simulink model "Space_Shuttle"  (R2023a)
settings: Solver=ode45  StartTime=0.0  StopTime=1000  RelTol=1e-4
undefined symbols (not defined in the file or in its folder): Earth, WGS84
libraries: simulink_extras x4, slpidlib x3, simulink x3, aerolibadyn x1, aerolibatmos2 x1, aerolib6dof2 x1
settings Model: PauseTimes=0  Creator=francesconuzzo  LastModifiedBy=francesconuzzo

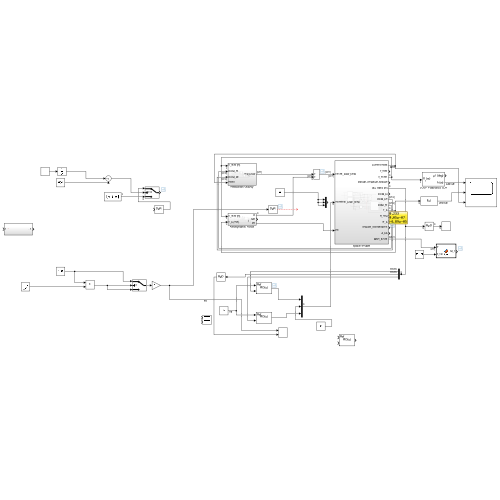
[thumbnail: Simulink's stored preview of the top-level diagram]
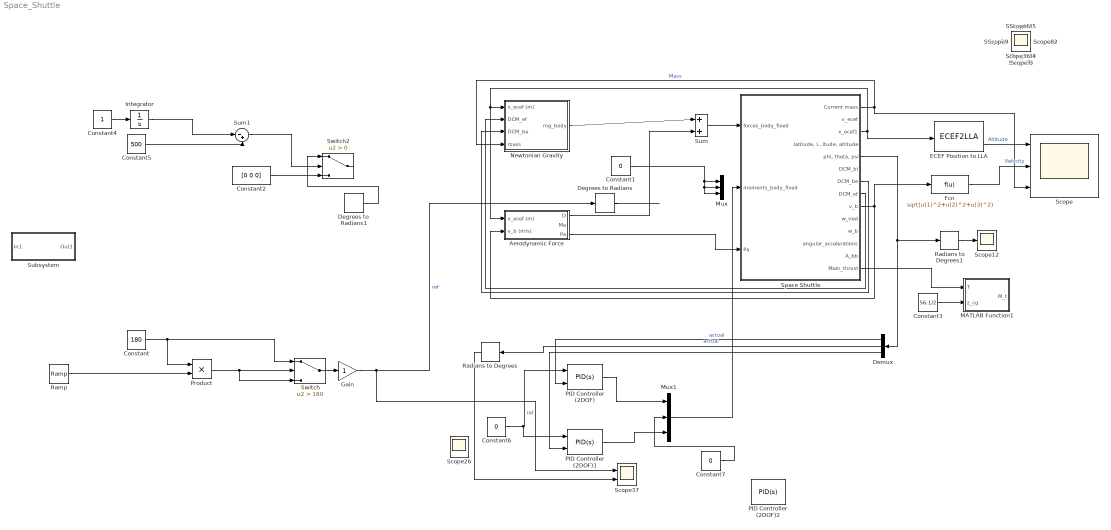
== system Space_Shuttle ==
  Aerodynamic Force : Subsystem
  Constant : Constant  Value=180
  Constant1 : Constant  Value=0
  Constant2 : Constant  Value=[0 0 0]
  Constant3 : Constant  Value=56.1/2
  Constant4 : Constant
  Constant5 : Constant  Value=500
  Constant6 : Constant  Value=0
  Constant7 : Constant  Value=0
  Degrees to Radians : simulink_extras/Transformations/Degrees to Radians
  Degrees to Radians1 : simulink_extras/Transformations/Degrees to Radians
  Demux : Demux  Outputs=3
  ECEF Position to LLA : ECEF2LLA
  Fcn : Fcn  Expr=sqrt(u(1)^2+u(2)^2+u(3)^2)
  Gain : Gain
  Integrator : Integrator
  MATLAB Function1 : MATLAB Function  TreatAsAtomicUnit=on
  Mux : Mux  Inputs=3
  Mux1 : Mux  Inputs=3
  Newtonian Gravity : Subsystem
  PID Controller (2DOF) : slpidlib/PID Controller (2DOF)  Controller=PID  Form=Parallel  TimeDomain=Continuous-time  UseExternalTs=off  SampleTime=-1  IntegratorMethod=Forward Euler  FilterMethod=Forward Euler  ControllerParametersSource=internal  P=1  I=0  UseKiTs=off  D=0  N=100  UseFilter=on  b=0  c=0  TunerSelectOption=Transfer Function Based (PID Tuner App)  InitialConditionSource=internal  InitialConditionForIntegrator=0  InitialConditionForFilter=0  DifferentiatorICPrevScaledInput=0  ExternalReset=none  TrackingMode=off  Kt=1  LimitOutput=off  SatLimitsSource=internal  UpperSaturationLimit=inf  LowerSaturationLimit=-inf  LinearizeAsGain=on  AntiWindupMode=none  Kb=1  LimitIntegrator=off  UpperIntegratorSaturationLimit=inf  LowerIntegratorSaturationLimit=-inf  POutMin=[]  POutMax=[]  IOutMin=[]  IOutMax=[]  DOutMin=[]  DOutMax=[]  NOutMin=[]  NOutMax=[]  bOutMin=[]  bOutMax=[]  cOutMin=[]  cOutMax=[]  SumOutMin=[]  SumOutMax=[]  SaturationOutMin=[]  SaturationOutMax=[]  PParamMin=[]  PParamMax=[]  IParamMin=[]  IParamMax=[]  DParamMin=[]  DParamMax=[]  NParamMin=[]  NParamMax=[]  bParamMin=[]  bParamMax=[]  cParamMin=[]  cParamMax=[]  KbParamMin=[]  KbParamMax=[]  KtParamMin=[]  KtParamMax=[]  KbOutMin=[]  KbOutMax=[]  KtOutMin=[]  KtOutMax=[]  IntegratorOutMin=[]  IntegratorOutMax=[]  FilterOutMin=[]  FilterOutMax=[]  SumI1OutMin=[]  SumI1OutMax=[]  SumI2OutMin=[]  SumI2OutMax=[]  SumI3OutMin=[]  SumI3OutMax=[]  SumI4OutMin=[]  SumI4OutMax=[]  SumDOutMin=[]  SumDOutMax=[]  Sum1OutMin=[]  Sum1OutMax=[]  Sum2OutMin=[]  Sum2OutMax=[]  Sum3OutMin=[]  Sum3OutMax=[]  DifferentiatorOutMin=[]  DifferentiatorOutMax=[]  FilterDiffOutCoefMin=[]  FilterDiffOutCoefMax=[]  ReciprocalOutMin=[]  ReciprocalOutMax=[]  SumDenOutMin=[]  SumDenOutMax=[]  SumNumOutMin=[]  SumNumOutMax=[]  DivideOutMin=[]  DivideOutMax=[]  UdiffTsProdOutMin=[]  UdiffTsProdOutMax=[]  NTsProdOutMin=[]  NTsProdOutMax=[]  UintegralTsProdOutMin=[]  UintegralTsProdOutMax=[]  UngainTsProdOutMin=[]  UngainTsProdOutMax=[]  ClampingZeroOutDataTypeStr=Inherit: Inherit via back propagation  ClampingZeroOutMin=[]  ClampingZeroOutMax=[]  FilterDenConstantOutDataTypeStr=Inherit: Inherit via back propagation  FilterDenConstantOutMin=[]  FilterDenConstantOutMax=[]  PCopyOutDataTypeStr=Inherit: Inherit via back propagation  PCopyOutMin=[]  PCopyOutMax=[]  NCopyOutDataTypeStr=Inherit: Inherit via back propagation  NCopyOutMin=[]  NCopyOutMax=[]  IntegratorContinuousStateAttributes=''  IntegratorStateMustResolveToSignalObject=off  IntegratorRTWStateStorageClass=Auto  FilterContinuousStateAttributes=''  FilterStateMustResolveToSignalObject=off  FilterRTWStateStorageClass=Auto  ParallelPVariant=InternalParameters  IdealPVariant=Disabled  IVariant=InternalParameters  DVariant=InternalParameters  bVariant=InternalParameters  cVariant=InternalParameters  IntegratorVariant=Continuous  SatVariant=Disabled  AWVariant=Passthrough  PCopyVariant=Disabled  TRVariant=Disabled  FdbkBlocksVariant=Forward  IdealPFdbkVariant=Disabled  SatFdbkVariant=Disabled  DerivativeFilterVariant=ContFilter  NVariant=InternalParameters  NCopyVariant=Disabled  FilterICVariant=InternalICsFilter  IntegratorICVariant=InternalICs  ExternalResetVariant=Disabled  TRSumVariant=Passthrough  SumFdbkVariant=Disabled  SumVariant=Sum_PID  TsampFilterVariant=InternalTs  TsampNgainVariant=Passthrough  TsampIntegralVariant=Disabled_SignalSpec  ExternalSaturationOutDataTypeStr=Inherit: Same as second input
  PID Controller (2DOF)1 : slpidlib/PID Controller (2DOF)  Controller=PID  Form=Parallel  TimeDomain=Continuous-time  UseExternalTs=off  SampleTime=-1  IntegratorMethod=Forward Euler  FilterMethod=Forward Euler  ControllerParametersSource=internal  P=1  I=0  UseKiTs=off  D=0  N=100  UseFilter=on  b=0  c=0  TunerSelectOption=Transfer Function Based (PID Tuner App)  InitialConditionSource=internal  InitialConditionForIntegrator=0  InitialConditionForFilter=0  DifferentiatorICPrevScaledInput=0  ExternalReset=none  TrackingMode=off  Kt=1  LimitOutput=off  SatLimitsSource=internal  UpperSaturationLimit=inf  LowerSaturationLimit=-inf  LinearizeAsGain=on  AntiWindupMode=none  Kb=1  LimitIntegrator=off  UpperIntegratorSaturationLimit=inf  LowerIntegratorSaturationLimit=-inf  POutMin=[]  POutMax=[]  IOutMin=[]  IOutMax=[]  DOutMin=[]  DOutMax=[]  NOutMin=[]  NOutMax=[]  bOutMin=[]  bOutMax=[]  cOutMin=[]  cOutMax=[]  SumOutMin=[]  SumOutMax=[]  SaturationOutMin=[]  SaturationOutMax=[]  PParamMin=[]  PParamMax=[]  IParamMin=[]  IParamMax=[]  DParamMin=[]  DParamMax=[]  NParamMin=[]  NParamMax=[]  bParamMin=[]  bParamMax=[]  cParamMin=[]  cParamMax=[]  KbParamMin=[]  KbParamMax=[]  KtParamMin=[]  KtParamMax=[]  KbOutMin=[]  KbOutMax=[]  KtOutMin=[]  KtOutMax=[]  IntegratorOutMin=[]  IntegratorOutMax=[]  FilterOutMin=[]  FilterOutMax=[]  SumI1OutMin=[]  SumI1OutMax=[]  SumI2OutMin=[]  SumI2OutMax=[]  SumI3OutMin=[]  SumI3OutMax=[]  SumI4OutMin=[]  SumI4OutMax=[]  SumDOutMin=[]  SumDOutMax=[]  Sum1OutMin=[]  Sum1OutMax=[]  Sum2OutMin=[]  Sum2OutMax=[]  Sum3OutMin=[]  Sum3OutMax=[]  DifferentiatorOutMin=[]  DifferentiatorOutMax=[]  FilterDiffOutCoefMin=[]  FilterDiffOutCoefMax=[]  ReciprocalOutMin=[]  ReciprocalOutMax=[]  SumDenOutMin=[]  SumDenOutMax=[]  SumNumOutMin=[]  SumNumOutMax=[]  DivideOutMin=[]  DivideOutMax=[]  UdiffTsProdOutMin=[]  UdiffTsProdOutMax=[]  NTsProdOutMin=[]  NTsProdOutMax=[]  UintegralTsProdOutMin=[]  UintegralTsProdOutMax=[]  UngainTsProdOutMin=[]  UngainTsProdOutMax=[]  ClampingZeroOutDataTypeStr=Inherit: Inherit via back propagation  ClampingZeroOutMin=[]  ClampingZeroOutMax=[]  FilterDenConstantOutDataTypeStr=Inherit: Inherit via back propagation  FilterDenConstantOutMin=[]  FilterDenConstantOutMax=[]  PCopyOutDataTypeStr=Inherit: Inherit via back propagation  PCopyOutMin=[]  PCopyOutMax=[]  NCopyOutDataTypeStr=Inherit: Inherit via back propagation  NCopyOutMin=[]  NCopyOutMax=[]  IntegratorContinuousStateAttributes=''  IntegratorStateMustResolveToSignalObject=off  IntegratorRTWStateStorageClass=Auto  FilterContinuousStateAttributes=''  FilterStateMustResolveToSignalObject=off  FilterRTWStateStorageClass=Auto  ParallelPVariant=InternalParameters  IdealPVariant=Disabled  IVariant=InternalParameters  DVariant=InternalParameters  bVariant=InternalParameters  cVariant=InternalParameters  IntegratorVariant=Continuous  SatVariant=Disabled  AWVariant=Passthrough  PCopyVariant=Disabled  TRVariant=Disabled  FdbkBlocksVariant=Forward  IdealPFdbkVariant=Disabled  SatFdbkVariant=Disabled  DerivativeFilterVariant=ContFilter  NVariant=InternalParameters  NCopyVariant=Disabled  FilterICVariant=InternalICsFilter  IntegratorICVariant=InternalICs  ExternalResetVariant=Disabled  TRSumVariant=Passthrough  SumFdbkVariant=Disabled  SumVariant=Sum_PID  TsampFilterVariant=InternalTs  TsampNgainVariant=Passthrough  TsampIntegralVariant=Disabled_SignalSpec  ExternalSaturationOutDataTypeStr=Inherit: Same as second input
  PID Controller (2DOF)2 : slpidlib/PID Controller (2DOF)  Controller=PID  Form=Parallel  TimeDomain=Continuous-time  UseExternalTs=off  SampleTime=-1  IntegratorMethod=Forward Euler  FilterMethod=Forward Euler  ControllerParametersSource=internal  P=1  I=1  UseKiTs=off  D=0  N=100  UseFilter=on  b=1  c=1  TunerSelectOption=Transfer Function Based (PID Tuner App)  InitialConditionSource=internal  InitialConditionForIntegrator=0  InitialConditionForFilter=0  DifferentiatorICPrevScaledInput=0  ExternalReset=none  TrackingMode=off  Kt=1  LimitOutput=off  SatLimitsSource=internal  UpperSaturationLimit=inf  LowerSaturationLimit=-inf  LinearizeAsGain=on  AntiWindupMode=none  Kb=1  LimitIntegrator=off  UpperIntegratorSaturationLimit=inf  LowerIntegratorSaturationLimit=-inf  POutMin=[]  POutMax=[]  IOutMin=[]  IOutMax=[]  DOutMin=[]  DOutMax=[]  NOutMin=[]  NOutMax=[]  bOutMin=[]  bOutMax=[]  cOutMin=[]  cOutMax=[]  SumOutMin=[]  SumOutMax=[]  SaturationOutMin=[]  SaturationOutMax=[]  PParamMin=[]  PParamMax=[]  IParamMin=[]  IParamMax=[]  DParamMin=[]  DParamMax=[]  NParamMin=[]  NParamMax=[]  bParamMin=[]  bParamMax=[]  cParamMin=[]  cParamMax=[]  KbParamMin=[]  KbParamMax=[]  KtParamMin=[]  KtParamMax=[]  KbOutMin=[]  KbOutMax=[]  KtOutMin=[]  KtOutMax=[]  IntegratorOutMin=[]  IntegratorOutMax=[]  FilterOutMin=[]  FilterOutMax=[]  SumI1OutMin=[]  SumI1OutMax=[]  SumI2OutMin=[]  SumI2OutMax=[]  SumI3OutMin=[]  SumI3OutMax=[]  SumI4OutMin=[]  SumI4OutMax=[]  SumDOutMin=[]  SumDOutMax=[]  Sum1OutMin=[]  Sum1OutMax=[]  Sum2OutMin=[]  Sum2OutMax=[]  Sum3OutMin=[]  Sum3OutMax=[]  DifferentiatorOutMin=[]  DifferentiatorOutMax=[]  FilterDiffOutCoefMin=[]  FilterDiffOutCoefMax=[]  ReciprocalOutMin=[]  ReciprocalOutMax=[]  SumDenOutMin=[]  SumDenOutMax=[]  SumNumOutMin=[]  SumNumOutMax=[]  DivideOutMin=[]  DivideOutMax=[]  UdiffTsProdOutMin=[]  UdiffTsProdOutMax=[]  NTsProdOutMin=[]  NTsProdOutMax=[]  UintegralTsProdOutMin=[]  UintegralTsProdOutMax=[]  UngainTsProdOutMin=[]  UngainTsProdOutMax=[]  ClampingZeroOutDataTypeStr=Inherit: Inherit via back propagation  ClampingZeroOutMin=[]  ClampingZeroOutMax=[]  FilterDenConstantOutDataTypeStr=Inherit: Inherit via back propagation  FilterDenConstantOutMin=[]  FilterDenConstantOutMax=[]  PCopyOutDataTypeStr=Inherit: Inherit via back propagation  PCopyOutMin=[]  PCopyOutMax=[]  NCopyOutDataTypeStr=Inherit: Inherit via back propagation  NCopyOutMin=[]  NCopyOutMax=[]  IntegratorContinuousStateAttributes=''  IntegratorStateMustResolveToSignalObject=off  IntegratorRTWStateStorageClass=Auto  FilterContinuousStateAttributes=''  FilterStateMustResolveToSignalObject=off  FilterRTWStateStorageClass=Auto  ParallelPVariant=InternalParameters  IdealPVariant=Disabled  IVariant=InternalParameters  DVariant=InternalParameters  bVariant=InternalParameters  cVariant=InternalParameters  IntegratorVariant=Continuous  SatVariant=Disabled  AWVariant=Passthrough  PCopyVariant=Disabled  TRVariant=Disabled  FdbkBlocksVariant=Forward  IdealPFdbkVariant=Disabled  SatFdbkVariant=Disabled  DerivativeFilterVariant=ContFilter  NVariant=InternalParameters  NCopyVariant=Disabled  FilterICVariant=InternalICsFilter  IntegratorICVariant=InternalICs  ExternalResetVariant=Disabled  TRSumVariant=Passthrough  SumFdbkVariant=Disabled  SumVariant=Sum_PID  TsampFilterVariant=InternalTs  TsampNgainVariant=Passthrough  TsampIntegralVariant=Disabled_SignalSpec  ExternalSaturationOutDataTypeStr=Inherit: Same as second input
  Product : Product
  Radians to Degrees : simulink_extras/Transformations/Radians to Degrees
  Radians to Degrees1 : simulink_extras/Transformations/Radians to Degrees
  Ramp : simulink/Sources/Ramp  slope=0.001  start=20  InitialOutput=0.5
  Scope : Scope  NumInputPorts=3
  Scope{1..25,27..36,38} (36 alike) : Scope
  Scope26 : Scope  NumInputPorts=2
  Scope37 : Scope  NumInputPorts=2
  Space Shuttle : Subsystem
  Subsystem : Subsystem
  Sum : Sum  Inputs=|++
  Sum1 : Sum  Inputs=|-+
  Switch : Switch  Criteria=u2 > Threshold  Threshold=180  SaturateOnIntegerOverflow=off  InputSameDT=off
  Switch2 : Switch  Criteria=u2 > Threshold  SaturateOnIntegerOverflow=off  InputSameDT=off
  wires:
  Space Shuttle/3(x_ecef1) -> ECEF Position to LLA/1, Aerodynamic Force/1(x_ecef (m)), Newtonian Gravity/1(x_ecef (m))
  Space Shuttle/9(v_b) -> Aerodynamic Force/2(v_b (m/s)), Fcn/1
  Space Shuttle/1(Current mass) -> Scope/3, Newtonian Gravity/4(mass)  "Mass"
  Space Shuttle/7(DCM_be) -> Newtonian Gravity/3(DCM_be)
  Space Shuttle/8(DCM_ef) -> Newtonian Gravity/2(DCM_ef)
  Sum/1 -> Space Shuttle/1(forces_body_fixed)
  Newtonian Gravity/1(mg_body) -> Sum/1
  Aerodynamic Force/1(D) -> Sum/2
  Aerodynamic Force/3(Pa) -> Space Shuttle/3(Pa)
  Space Shuttle/5("phi, theta, psi") -> Demux/1, Radians to Degrees1/1
  ECEF Position to LLA/2 -> Scope/1  "Altitude"
  Fcn/1 -> Scope/2  "Velocity"
  Radians to Degrees1/1 -> Scope12/1
  Constant4/1 -> Integrator/1
  Sum1/1 -> Switch2/2
  Integrator/1 -> Sum1/1
  Constant5/1 -> Sum1/2
  Constant/1 -> Product/1, Switch/1
  Product/1 -> Switch/2, Switch/3
  Constant2/1 -> Switch2/3
  Degrees to Radians1/1 -> Switch2/1
  Ramp/1 -> Product/2
  Space Shuttle/14(Main_thrust) -> MATLAB Function1/1(T)
  Constant3/1 -> MATLAB Function1/2(z_cg)
  Switch/1 -> Gain/1
  Constant1/1 -> Mux/2, Mux/3, Mux/1
  Degrees to Radians/1 -> ?
  Demux/1 -> PID Controller (2DOF)/2  "actual"
  Demux/2 -> Radians to Degrees/1  "actual"
  Demux/3 -> PID Controller (2DOF)1/2
  Constant6/1 -> PID Controller (2DOF)1/1, PID Controller (2DOF)/1  "ref"
  Gain/1 -> Scope37/1, Degrees to Radians/1  "ref"
  PID Controller (2DOF)/1 -> Mux1/1
  PID Controller (2DOF)1/1 -> Mux1/3
  Mux1/1 -> Space Shuttle/2(moments_body_fixed)
  Constant7/1 -> Mux1/2
  Radians to Degrees/1 -> Scope37/2

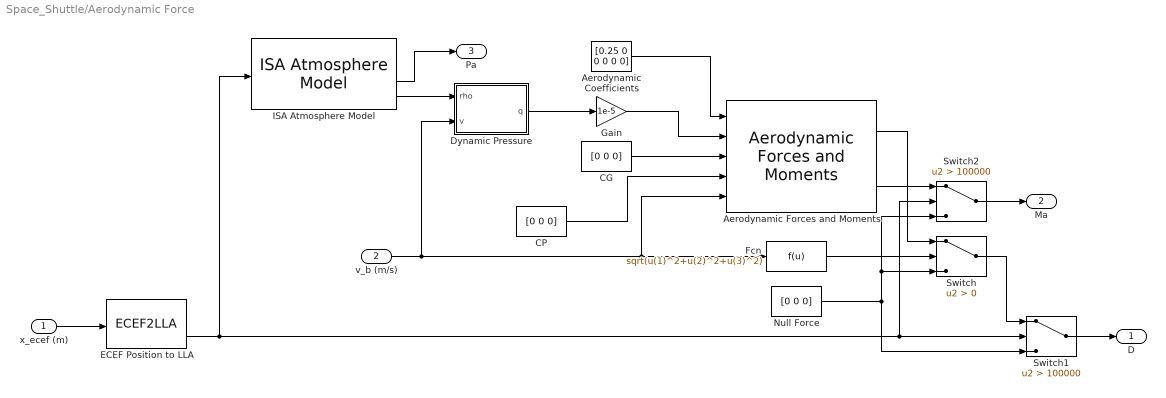
== system Space_Shuttle/Aerodynamic Force ==
  x_ecef (m) : Inport
  v_b (m/s) : Inport  Port=2
  "Aerodynamic Forces and Moments " : aerolibadyn/Aerodynamic Forces and Moments   inputAxes=Wind  outputForceAxes=Body  outputMomentAxes=Body  S=0.78  b=1  cbar=56.1
  Aerodynamic Coefficients : Constant  Value=[0.25 0 0 0 0 0]
  CG : Constant  Value=[0 0 0]
  CP : Constant  Value=[0 0 0]
  Dynamic Pressure : MATLAB Function  TreatAsAtomicUnit=on
  ECEF Position to LLA : ECEF2LLA
  Fcn : Fcn  Expr=sqrt(u(1)^2+u(2)^2+u(3)^2)
  Gain : Gain  Gain=1e-5
  ISA Atmosphere Model : aerolibatmos2/ISA Atmosphere Model  custom=off  g=9.80665  gamma=1.4  R=287.0531  L=0.0065  h_trop=11000  h_strat=20000  rho0=1.225  P0=101325  T0=288.15  h0=0
  Null Force : Constant  Value=[0 0 0]
  Switch : Switch  Criteria=u2 > Threshold  SaturateOnIntegerOverflow=off  InputSameDT=off
  Switch1 : Switch  Criteria=u2 > Threshold  Threshold=100000  SaturateOnIntegerOverflow=off  InputSameDT=off
  Switch2 : Switch  Criteria=u2 > Threshold  Threshold=100000  SaturateOnIntegerOverflow=off  InputSameDT=off
  D : Outport
  Ma : Outport  Port=2
  Pa : Outport  Port=3
  wires:
  Switch2/1 -> Ma/1
  Null Force/1 -> Switch/3, Switch2/3, Switch1/3
  Fcn/1 -> Switch/2
  "Aerodynamic Forces and Moments "/2 -> Switch2/1
  CG/1 -> "Aerodynamic Forces and Moments "/3
  Gain/1 -> "Aerodynamic Forces and Moments "/2
  Aerodynamic Coefficients/1 -> "Aerodynamic Forces and Moments "/1
  Dynamic Pressure/1(q) -> Gain/1
  v_b (m/s)/1 -> Fcn/1, "Aerodynamic Forces and Moments "/5, Dynamic Pressure/2(v)
  CP/1 -> "Aerodynamic Forces and Moments "/4
  ISA Atmosphere Model/3 -> Pa/1
  ECEF Position to LLA/2 -> Switch2/2, Switch1/2, ISA Atmosphere Model/1
  ISA Atmosphere Model/4 -> Dynamic Pressure/1(rho)
  "Aerodynamic Forces and Moments "/1 -> Switch/1
  Switch1/1 -> D/1
  Switch/1 -> Switch1/1
  x_ecef (m)/1 -> ECEF Position to LLA/1

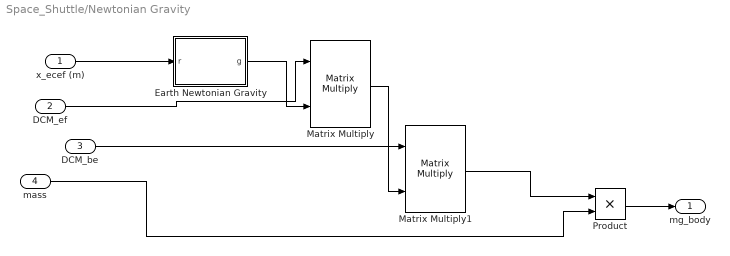
== system Space_Shuttle/Newtonian Gravity ==
  x_ecef (m) : Inport
  DCM_ef : Inport  Port=2
  DCM_be : Inport  Port=3
  mass : Inport  Port=4
  Earth Newtonian Gravity : MATLAB Function  TreatAsAtomicUnit=on
  Matrix Multiply : Product  Multiplication=Matrix(*)
  Matrix Multiply1 : Product  Multiplication=Matrix(*)
  Product : Product
  mg_body : Outport
  wires:
  Earth Newtonian Gravity/1(g) -> Matrix Multiply/2
  DCM_ef/1 -> Matrix Multiply/1
  x_ecef (m)/1 -> Earth Newtonian Gravity/1(r)
  Matrix Multiply/1 -> Matrix Multiply1/2
  DCM_be/1 -> Matrix Multiply1/1
  Matrix Multiply1/1 -> Product/1
  mass/1 -> Product/2
  Product/1 -> mg_body/1

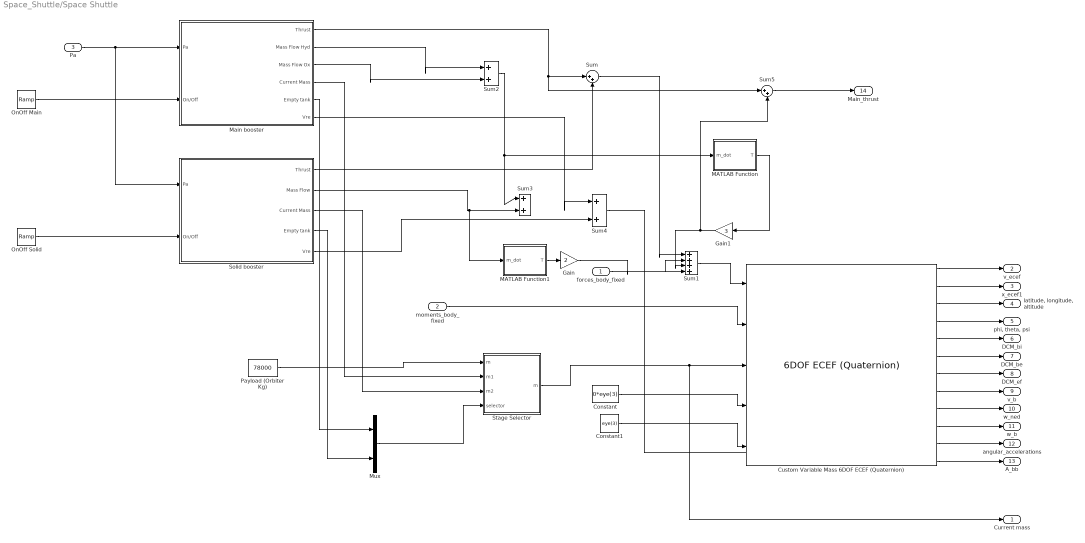
== system Space_Shuttle/Space Shuttle ==
  forces_body_fixed : Inport
  moments_body_fixed : Inport  Port=2
  Pa : Inport  Port=3
  Constant : Constant  Value=0*eye(3)
  Constant1 : Constant  Value=eye(3)
  Custom Variable Mass 6DOF ECEF (Quaternion) : aerolib6dof2/6DOF ECEF (Quaternion)  units=Metric (MKS)  mtype=Custom Variable  xg_0=[5.24 -52.77 110]  Vm_0=[0 0 0]  eul_0=[0 -pi/2 0]  pm_0=[0 0 0]  mass_0=1.0  mass_e=0.5  mass_f=2.0  inertia=eye(3)  inertia_e=eye(3)  inertia_f=2*eye(3)  vre_flag=off  abi_flag=off  ptype=Earth (WGS84)  R=6378137  F=1/298.257223563  w_E=7292115e-11  angle_in=Internal  LG0=0  quat_statename=''  pm_statename=''  Vm_statename=''  posECEF_statename=''  posECI_statename=''  LG_statename=''  mass_statename=''
      settings: LibrarySourceBlock=|
      | aerolib6dof2/Custom Variable Mass 6DOF
      | ECEF (Quaternion)
  Gain : Gain  Gain=2
  Gain1 : Gain  Gain=3
  MATLAB Function : MATLAB Function  TreatAsAtomicUnit=on
  MATLAB Function1 : MATLAB Function  TreatAsAtomicUnit=on
  Main booster : Subsystem
  Mux : Mux  Inputs=2
  OnOff Main : simulink/Sources/Ramp  slope=1  start=0  InitialOutput=0
  OnOff Solid : simulink/Sources/Ramp  slope=1  start=0  InitialOutput=0
  Payload (Orbiter Kg) : Constant  Value=78000
  Solid booster : Subsystem
  Stage Selector : MATLAB Function  TreatAsAtomicUnit=on
  Sum{,2..5} (5 alike) : Sum  Inputs=|++
  Sum1 : Sum  Inputs=|++++
  Current mass : Outport
  v_ecef : Outport  Port=2
  x_ecef1 : Outport  Port=3
  "latitude, longitude, altitude" : Outport  Port=4
  "phi, theta, psi" : Outport  Port=5
  DCM_bi : Outport  Port=6
  DCM_be : Outport  Port=7
  DCM_ef : Outport  Port=8
  v_b : Outport  Port=9
  w_ned : Outport  Port=10
  w_b : Outport  Port=11
  angular_accelerations : Outport  Port=12
  A_bb : Outport  Port=13
  Main_thrust : Outport  Port=14
  wires:
  Custom Variable Mass 6DOF ECEF (Quaternion)/1 -> v_ecef/1
  Custom Variable Mass 6DOF ECEF (Quaternion)/2 -> x_ecef1/1
  Custom Variable Mass 6DOF ECEF (Quaternion)/3 -> "latitude, longitude, altitude"/1
  Custom Variable Mass 6DOF ECEF (Quaternion)/4 -> "phi, theta, psi"/1
  Custom Variable Mass 6DOF ECEF (Quaternion)/5 -> DCM_bi/1
  Custom Variable Mass 6DOF ECEF (Quaternion)/6 -> DCM_be/1
  Custom Variable Mass 6DOF ECEF (Quaternion)/7 -> DCM_ef/1
  Custom Variable Mass 6DOF ECEF (Quaternion)/8 -> v_b/1
  Custom Variable Mass 6DOF ECEF (Quaternion)/9 -> w_ned/1
  Custom Variable Mass 6DOF ECEF (Quaternion)/10 -> w_b/1
  Custom Variable Mass 6DOF ECEF (Quaternion)/11 -> angular_accelerations/1
  Custom Variable Mass 6DOF ECEF (Quaternion)/12 -> A_bb/1
  moments_body_fixed/1 -> Custom Variable Mass 6DOF ECEF (Quaternion)/2
  Constant/1 -> Custom Variable Mass 6DOF ECEF (Quaternion)/4
  Constant1/1 -> Custom Variable Mass 6DOF ECEF (Quaternion)/5
  Main booster/1(Thrust) -> Sum5/1, Sum/1
  Solid booster/1(Thrust) -> Sum/2
  Sum/1 -> Sum1/1
  forces_body_fixed/1 -> Sum1/2
  Main booster/2(Mass Flow Hyd) -> Sum2/1
  Main booster/3(Mass Flow Ox) -> Sum2/2
  Sum2/1 -> MATLAB Function/1(m_dot), Sum3/1
  Solid booster/2("Mass Flow ") -> MATLAB Function1/1(m_dot), Sum3/2
  Main booster/6(Vre) -> Sum4/1
  Solid booster/5(Vre) -> Sum4/2
  Sum4/1 -> ?
  Stage Selector/1(m) -> Current mass/1, Custom Variable Mass 6DOF ECEF (Quaternion)/3
  Main booster/4(Current Mass) -> Stage Selector/2(m1)
  Solid booster/3(Current Mass) -> Stage Selector/3(m2)
  Mux/1 -> Stage Selector/4(selector)
  Payload (Orbiter Kg)/1 -> Stage Selector/1("m ")
  Main booster/5(Empty tank) -> Mux/1
  Solid booster/4(Empty tank) -> Mux/2
  Pa/1 -> Solid booster/1(Pa), Main booster/1(Pa)
  OnOff Main/1 -> Main booster/2(On/Off)
  OnOff Solid/1 -> Solid booster/2(On/Off)
  Sum1/1 -> Custom Variable Mass 6DOF ECEF (Quaternion)/1
  MATLAB Function/1(T) -> Gain1/1
  MATLAB Function1/1(T) -> Gain/1
  Gain/1 -> Sum1/4
  Gain1/1 -> Sum1/3, Sum5/2
  Sum5/1 -> Main_thrust/1

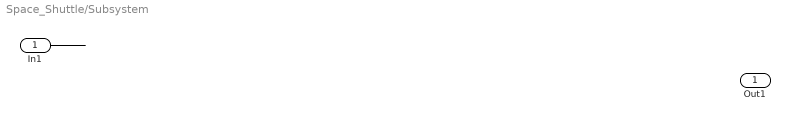
== system Space_Shuttle/Subsystem ==
  In1 : Inport
  Out1 : Outport
  wires:
  In1/1 -> ?

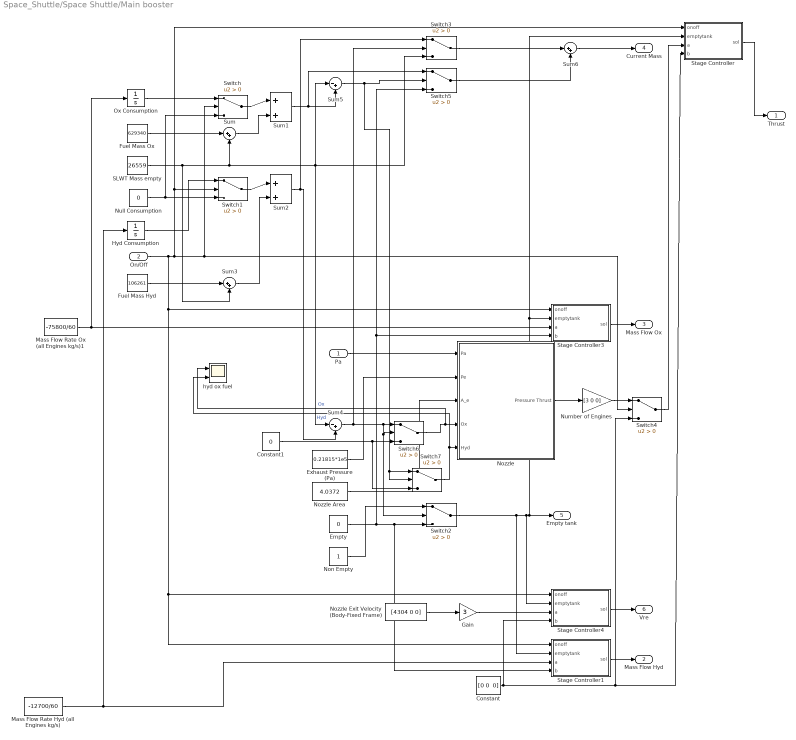
== system Space_Shuttle/Space Shuttle/Main booster ==
  Pa : Inport
  On/Off : Inport  Port=2
  Constant : Constant  Value="[0 0  0]"
  Constant1 : Constant  Value=0
  Empty : Constant  Value=0
  Exhaust Pressure (Pa) : Constant  Value=0.21815*1e5
  Fuel Mass Hyd : Constant  Value=106261
  Fuel Mass Ox : Constant  Value=629340
  Gain : Gain  Gain=3
  Hyd Consumption : Integrator
  Mass Flow Rate Hyd (all Engines kg/s) : Constant  Value=-12700/60
  Mass Flow Rate Ox (all Engines kg/s)1 : Constant  Value=-75800/60
  Non Empty : Constant
  Nozzle : Subsystem
  Nozzle Area : Constant  Value=4.0372
  Nozzle Exit Velocity (Body-Fixed Frame) : Constant  Value=[4304 0 0]
  Null Consumption : Constant  Value=0
  Number of Engines : Gain  Gain=[3 0 0]
  Ox Consumption : Integrator
  SLWT Mass empty : Constant  Value=26559
  Stage Controller : MATLAB Function  TreatAsAtomicUnit=on
  Stage Controller1 : MATLAB Function  TreatAsAtomicUnit=on
  Stage Controller3 : MATLAB Function  TreatAsAtomicUnit=on
  Stage Controller4 : MATLAB Function  TreatAsAtomicUnit=on
  Sum{,1..3,6} (5 alike) : Sum  Inputs=|++
  Sum4 : Sum  Inputs=|-+
  Sum5 : Sum  Inputs=|-+
  Switch{,1..7} (8 alike) : Switch  Criteria=u2 > Threshold  SaturateOnIntegerOverflow=off  InputSameDT=off
  hyd ox fuel : Scope  NumInputPorts=2
  Thrust : Outport
  Mass Flow Hyd : Outport  Port=2
  Mass Flow Ox : Outport  Port=3
  Current Mass : Outport  Port=4
  Empty tank : Outport  Port=5
  Vre : Outport  Port=6
  wires:
  Switch4/1 -> Stage Controller/3(a)
  Stage Controller4/1(sol) -> Vre/1
  Number of Engines/1 -> Switch4/1
  Stage Controller1/1(sol) -> Mass Flow Hyd/1
  Stage Controller3/1(sol) -> Mass Flow Ox/1
  Nozzle Exit Velocity (Body-Fixed Frame)/1 -> Gain/1
  Nozzle/1(Pressure Thrust) -> Number of Engines/1
  Ox Consumption/1 -> Switch/1
  Nozzle Area/1 -> Nozzle/3(A_e)
  Sum6/1 -> Current Mass/1
  Switch3/1 -> Sum6/1
  Switch1/1 -> Sum2/1
  Exhaust Pressure (Pa)/1 -> Nozzle/2(Pe)
  Mass Flow Rate Hyd (all Engines kg/s)/1 -> Hyd Consumption/1, Stage Controller1/3(a)
  Pa/1 -> Nozzle/1(Pa)
  Sum5/1 -> Switch7/2, Switch7/1, Switch5/2
  Sum2/1 -> Switch3/1, Sum4/2
  Constant/1 -> Switch4/3, Stage Controller/4(b), Stage Controller4/4(b)
  Sum4/1 -> Switch6/2, Switch2/2, Switch6/1, Switch3/2
  Sum1/1 -> Switch5/1, Sum5/2
  Sum3/1 -> Sum2/2
  On/Off/1 -> Stage Controller1/1(onoff), Stage Controller4/1(onoff), Stage Controller3/1(onoff), Switch/2, Switch4/2, Switch1/2, Stage Controller/1(onoff)
  Fuel Mass Hyd/1 -> Sum3/1
  Fuel Mass Ox/1 -> Sum/1
  Sum/1 -> Sum1/2
  Switch/1 -> Sum1/1
  Non Empty/1 -> Switch2/1
  Switch5/1 -> Sum6/2
  Hyd Consumption/1 -> Switch1/1
  Switch2/1 -> Stage Controller3/2(emptytank), Stage Controller/2(emptytank), Empty tank/1, Stage Controller4/2(emptytank), Stage Controller1/2(emptytank)
  Empty/1 -> Switch2/3, Stage Controller1/4(b), Switch5/3, Stage Controller3/4(b)
  Null Consumption/1 -> Switch1/3, Switch/3
  SLWT Mass empty/1 -> Sum5/1, Switch3/3, Sum4/1, Sum/2, Sum3/2
  Mass Flow Rate Ox (all Engines kg/s)1/1 -> Ox Consumption/1, Stage Controller3/3(a)
  Constant1/1 -> Switch7/3, Switch6/3
  Switch7/1 -> hyd ox fuel/2, Nozzle/5(Hyd)  "Hyd"
  Switch6/1 -> hyd ox fuel/1, Nozzle/4(Ox)  "Ox"
  Stage Controller/1(sol) -> Thrust/1
  Gain/1 -> Stage Controller4/3(a)

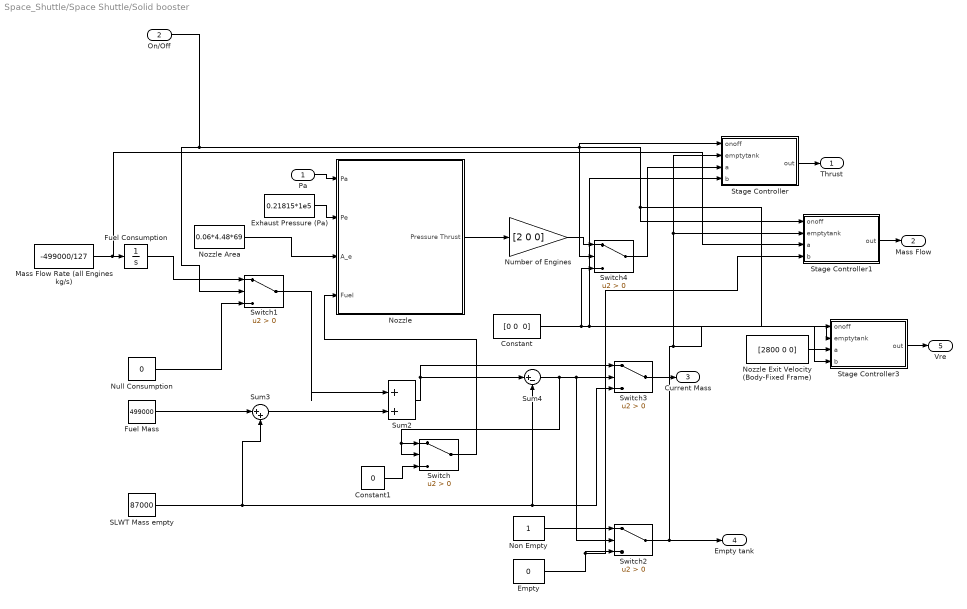
== system Space_Shuttle/Space Shuttle/Solid booster ==
  Pa : Inport
  On/Off : Inport  Port=2
  Constant : Constant  Value="[0 0  0]"
  Constant1 : Constant  Value=0
  Empty : Constant  Value=0
  Exhaust Pressure (Pa) : Constant  Value=0.21815*1e5
  Fuel Consumption : Integrator
  "Fuel Mass " : Constant  Value=499000
  Mass Flow Rate (all Engines kg/s) : Constant  Value=-499000/127
  Non Empty : Constant
  Nozzle : Subsystem
  Nozzle Area : Constant  Value=0.06*4.48*69
  Nozzle Exit Velocity (Body-Fixed Frame) : Constant  Value=[2800 0 0]
  Null Consumption : Constant  Value=0
  Number of Engines : Gain  Gain=[2 0 0]
  SLWT Mass empty : Constant  Value=87000
  Stage Controller : MATLAB Function  TreatAsAtomicUnit=on
  Stage Controller1 : MATLAB Function  TreatAsAtomicUnit=on
  Stage Controller3 : MATLAB Function  TreatAsAtomicUnit=on
  Sum2 : Sum  Inputs=|++
  Sum3 : Sum  Inputs=|++
  Sum4 : Sum  Inputs=|+-
  Switch{,1..4} (5 alike) : Switch  Criteria=u2 > Threshold  SaturateOnIntegerOverflow=off  InputSameDT=off
  Thrust : Outport
  "Mass Flow " : Outport  Port=2
  Current Mass : Outport  Port=3
  Empty tank : Outport  Port=4
  Vre : Outport  Port=5
  wires:
  Switch2/1 -> Stage Controller3/2(emptytank), Stage Controller/2(emptytank), Stage Controller1/2(emptytank), Empty tank/1
  Sum4/1 -> Switch/1, Switch/2, Switch3/2, Switch2/2
  Sum2/1 -> Sum4/1, Switch3/1
  Nozzle/1(Pressure Thrust) -> Number of Engines/1
  Sum3/1 -> Sum2/2
  Switch1/1 -> Sum2/1
  Nozzle Area/1 -> Nozzle/3(A_e)
  Exhaust Pressure (Pa)/1 -> Nozzle/2(Pe)
  Pa/1 -> Nozzle/1(Pa)
  SLWT Mass empty/1 -> Sum4/2, Switch3/3, Sum3/2
  "Fuel Mass "/1 -> Sum3/1
  Empty/1 -> Stage Controller1/4(b), Switch2/3
  Null Consumption/1 -> Switch1/3
  Mass Flow Rate (all Engines kg/s)/1 -> Stage Controller1/3(a), Fuel Consumption/1
  Non Empty/1 -> Switch2/1
  On/Off/1 -> Stage Controller1/1(onoff), Stage Controller3/1(onoff), Stage Controller/1(onoff), Switch4/2, Switch1/2
  Fuel Consumption/1 -> Switch1/1
  Number of Engines/1 -> Switch4/1
  Constant/1 -> Stage Controller/4(b), Stage Controller3/4(b), Switch4/3
  Switch4/1 -> Stage Controller/3(a)
  Nozzle Exit Velocity (Body-Fixed Frame)/1 -> Stage Controller3/3(a)
  Switch3/1 -> Current Mass/1
  Stage Controller/1(out) -> Thrust/1
  Stage Controller1/1(out) -> "Mass Flow "/1
  Stage Controller3/1(out) -> Vre/1
  Constant1/1 -> Switch/3
  Switch/1 -> Nozzle/4(Fuel)

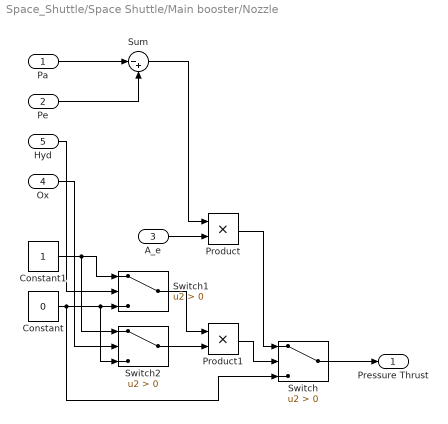
== system Space_Shuttle/Space Shuttle/Main booster/Nozzle ==
  Pa : Inport
  Pe : Inport  Port=2
  A_e : Inport  Port=3
  Ox : Inport  Port=4
  Hyd : Inport  Port=5
  Constant : Constant  Value=0
  Constant1 : Constant
  Product : Product
  Product1 : Product
  Sum : Sum  Inputs=|-+
  Switch : Switch  Criteria=u2 > Threshold  SaturateOnIntegerOverflow=off  InputSameDT=off
  Switch1 : Switch  Criteria=u2 > Threshold  SaturateOnIntegerOverflow=off  InputSameDT=off
  Switch2 : Switch  Criteria=u2 > Threshold  SaturateOnIntegerOverflow=off  InputSameDT=off
  Pressure Thrust : Outport
  wires:
  Switch/1 -> Pressure Thrust/1
  Product1/1 -> Switch/2
  Product/1 -> Switch/1
  A_e/1 -> Product/2
  Sum/1 -> Product/1
  Switch1/1 -> Product1/1
  Pe/1 -> Sum/2
  Constant/1 -> Switch2/3, Switch1/3, Switch/3
  Ox/1 -> Switch2/2
  Switch2/1 -> Product1/2
  Pa/1 -> Sum/1
  Constant1/1 -> Switch2/1, Switch1/1
  Hyd/1 -> Switch1/2

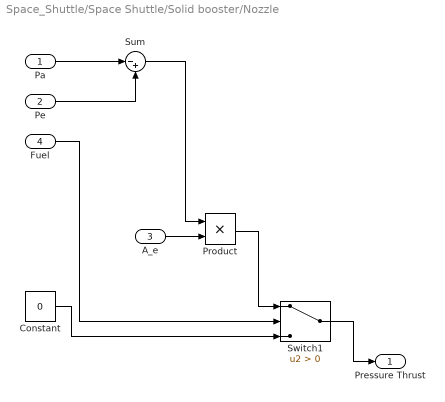
== system Space_Shuttle/Space Shuttle/Solid booster/Nozzle ==
  Pa : Inport
  Pe : Inport  Port=2
  A_e : Inport  Port=3
  Fuel : Inport  Port=4
  Constant : Constant  Value=0
  Product : Product
  Sum : Sum  Inputs=|-+
  Switch1 : Switch  Criteria=u2 > Threshold  SaturateOnIntegerOverflow=off  InputSameDT=off
  Pressure Thrust : Outport
  wires:
  A_e/1 -> Product/2
  Sum/1 -> Product/1
  Pe/1 -> Sum/2
  Constant/1 -> Switch1/3
  Pa/1 -> Sum/1
  Fuel/1 -> Switch1/2
  Product/1 -> Switch1/1
  Switch1/1 -> Pressure Thrust/1

== matlab function Space_Shuttle/Space Shuttle/Main booster/Stage Controller1 ==
  data: onoff input; sol output; emptytank input; a input; b input
function sol = fcn(onoff,emptytank,a,b)
if onoff >= 1 && emptytank == 1
    sol = a;
else 
    sol = b;
end

== matlab function Space_Shuttle/Space Shuttle/Main booster/Stage Controller4 ==
  data: onoff input; sol output; emptytank input; a input; b input
function sol = fcn(onoff,emptytank,a,b)
if onoff >= 1 && emptytank == 1
    sol = a;
else 
    sol = b;
end

== matlab function Space_Shuttle/Space Shuttle/MATLAB Function1 ==
  data: m_dot input; T output
function T = fcn(m_dot)
Isp = 298; g = 9.81;
T = Isp*m_dot*g;

== matlab function Space_Shuttle/MATLAB Function1 ==
  data: T input; M_t output; z_cg input
function M_t = fcn(T,z_cg)
M_t = zeros(3,1);
M_t(1) = z_cg*T(2); 
M_t(2) = -z_cg*T(1);
M_t(3) = 0;

== matlab function Space_Shuttle/Space Shuttle/Main booster/Stage Controller ==
  data: onoff input; sol output; emptytank input; a input; b input
function sol = fcn(onoff,emptytank,a,b)
if onoff >= 1 && emptytank == 1
    sol = a;
else 
    sol = b;
end

== matlab function Space_Shuttle/Space Shuttle/MATLAB Function ==
  data: m_dot input; T output
function T = fcn(m_dot)
Isp = 452; g = 9.81;
T = Isp*m_dot*g;

== matlab function Space_Shuttle/Space Shuttle/Main booster/Stage Controller3 ==
  data: onoff input; sol output; emptytank input; a input; b input
function sol = fcn(onoff,emptytank,a,b)
if onoff >= 1 && emptytank == 1
    sol = a;
else 
    sol = b;
end

== matlab function Space_Shuttle/Space Shuttle/Solid booster/Stage Controller ==
  data: onoff input; out output; emptytank input; a input; b input
function out = fcn(onoff,emptytank,a,b)
if onoff >= 1 && emptytank == 1
    out = a;
else 
    out = b;
end

== matlab function Space_Shuttle/Space Shuttle/Solid booster/Stage Controller1 ==
  data: onoff input; out output; emptytank input; a input; b input
function out = fcn(onoff,emptytank,a,b)
if onoff >= 1 && emptytank == 1
    out = a;
else 
    out = b;
end

== matlab function Space_Shuttle/Space Shuttle/Stage Selector ==
  data: m input; m1 input; m output; m2 input; selector input
function m = fcn(m,m1,m2,selector)
if selector(1) == 1
    m = m + m1;
end
if selector(2) == 1
    m = m + m2;
end

== matlab function Space_Shuttle/Space Shuttle/Solid booster/Stage Controller3 ==
  data: onoff input; out output; emptytank input; a input; b input
function out = fcn(onoff,emptytank,a,b)
if onoff >= 1 && emptytank == 1
    out = a;
else 
    out = b;
end

== matlab function Space_Shuttle/Newtonian Gravity/Earth Newtonian Gravity ==
  data: r input; g output
function g = fcn(r)
mu = 3.986004418e14;
g = (-mu/norm(r)^3).*r;

== matlab function Space_Shuttle/Aerodynamic Force/Dynamic Pressure ==
  data: rho input; q output; v input
function q = fcn(rho, v)
q = 0.5*rho*dot(v,v);
